simulink model "subVehicle"  (R2016a)
settings: Solver=VariableStepAuto  StartTime=0.0  StopTime=10.0  RelTol=1e-3
settings Model: Creator=Josef  LastModifiedBy=Josef
settings GRTTargetCC: GeneratePreprocessorConditionals=Use local settings

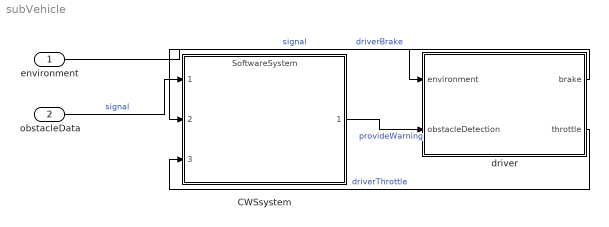
== system subVehicle ==
  environment : Inport
      settings: AttributesFormatString=signal
  obstacleData : Inport  Port=2
      settings: AttributesFormatString=signal
  CWSsystem : ModelReference  ModelNameDialog=SoftwareSystem  SimulationMode=Normal  ModelReferenceVersion=1.16
  driver : Subsystem
  wires:
  CWSsystem/1 -> driver/2(obstacleDetection)  "provideWarning"
  driver/1(brake) -> CWSsystem/2  "driverBrake"
  driver/2(throttle) -> CWSsystem/3  "driverThrottle"
  environment/1 -> driver/1(environment)  "signal"
  obstacleData/1 -> CWSsystem/1  "signal"

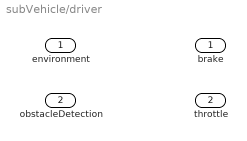
== system subVehicle/driver ==
  environment : Inport
      settings: AttributesFormatString=signal
  obstacleDetection : Inport  Port=2
      settings: AttributesFormatString=provideWarning
  brake : Outport
      settings: AttributesFormatString=driverBrake
  throttle : Outport  Port=2
      settings: AttributesFormatString=driverThrottle
